simulink model "DENEY3"  (R2023b)
settings: Solver=VariableStepAuto  StartTime=0.0  StopTime=10.0  RelTol=1e-3
libraries: dspfdesign x1, commrandsrc3 x1
settings Model: Creator=fatih  LastModifiedBy=fatih

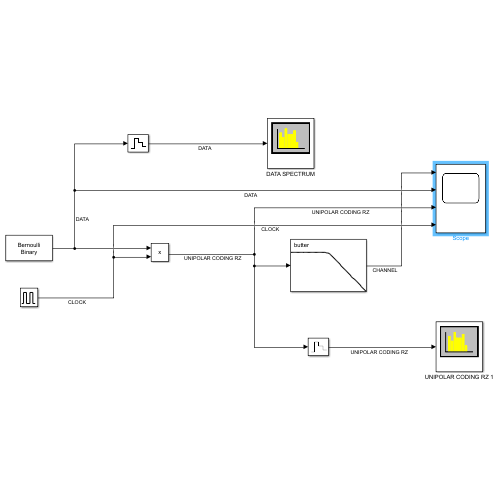
[thumbnail: Simulink's stored preview of the top-level diagram]
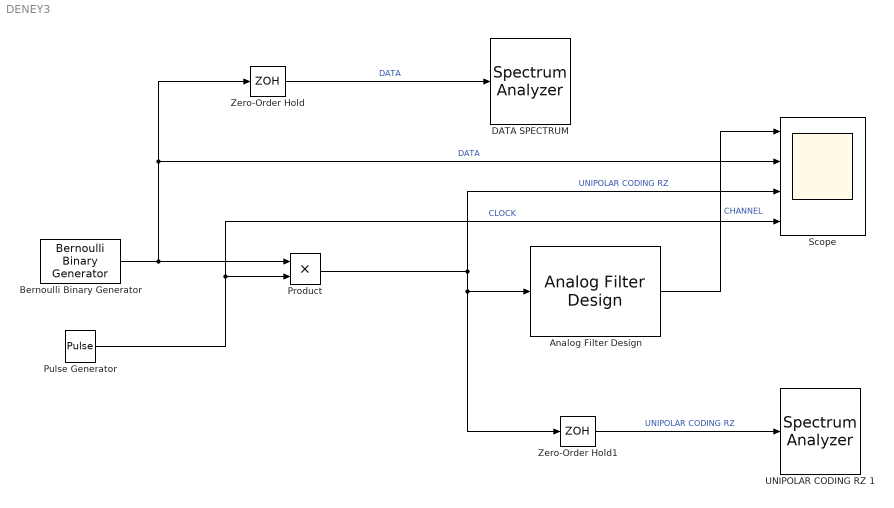
== system DENEY3 ==
  Analog Filter Design : dspfdesign/Analog Filter Design  method=Butterworth  filttype=Lowpass  N=8  Wlo=30  Whi=80  Rp=2  Rs=40
  Bernoulli Binary Generator : commrandsrc3/Bernoulli Binary Generator  ProbabilityOfZero=0.5  SeedSource=Auto  Seed=0  SampleTime=1  SamplesPerFrame=1  OutputDataType=double  SimulateUsing=Interpreted execution
  DATA SPECTRUM : SpectrumAnalyzer  Tag=DATA SPECTRUM  WindowPosition=[854.000000,66.000000,800.000000,407.000000,]  ScopeFrameLocation=window  Method=Welch  SampleRateSource=Property  SampleRate=44.1e3  FrequencySpan=Start and stop frequencies  StartFrequency=20  StopFrequency=20e3  YLimits=[-75.8908445,41.51853161]  SelectedToolstripTab=spectrumAnalyzerToolstrip.spectrumTab
  Product : Product
  Pulse Generator : DiscretePulseGenerator  Description=CLOCK  PulseType=Time based  Amplitude=5  Period=1/125  PulseWidth=50  VectorParams1D=off
  Scope : Scope  NumInputPorts=4
  UNIPOLAR CODING RZ 1 : SpectrumAnalyzer  WindowPosition=[541.000000,242.000000,800.000000,500.000000,]  ScopeFrameLocation=window  Method=Welch  SampleRateSource=Property  SampleRate=44.1e3  FrequencySpan=Start and stop frequencies  StartFrequency=20  StopFrequency=20e3  YLimits=[-67.98632576,49.48862167]  SelectedToolstripTab=spectrumAnalyzerToolstrip.spectrumTab
  Zero-Order Hold : ZeroOrderHold  SampleTime=1/100000
  Zero-Order Hold1 : ZeroOrderHold  SampleTime=1/100000
  wires:
  Bernoulli Binary Generator/1 -> Scope/2, Zero-Order Hold/1, Product/1  "DATA"
  Pulse Generator/1 -> Scope/4, Product/2  "CLOCK"
  Analog Filter Design/1 -> Scope/1  "CHANNEL"
  Product/1 -> Zero-Order Hold1/1, Analog Filter Design/1, Scope/3  "UNIPOLAR CODING RZ"
  Zero-Order Hold/1 -> DATA SPECTRUM/1  "DATA"
  Zero-Order Hold1/1 -> UNIPOLAR CODING RZ 1/1  "UNIPOLAR CODING RZ"
